simulink model "BC_DC_MotorModel"  (R2022b)
settings: Solver=VariableStepAuto  StartTime=0.0  StopTime=10  RelTol=1e-3
undefined symbols (not defined in the file): b, J, Ke, Kt, L, R
settings Model: Creator=altay  LastModifiedBy=altay

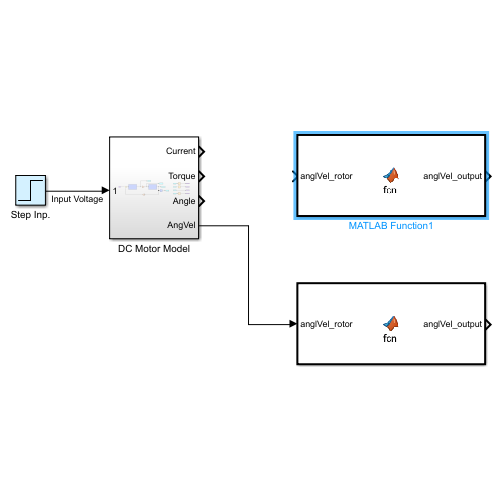
[thumbnail: Simulink's stored preview of the top-level diagram]
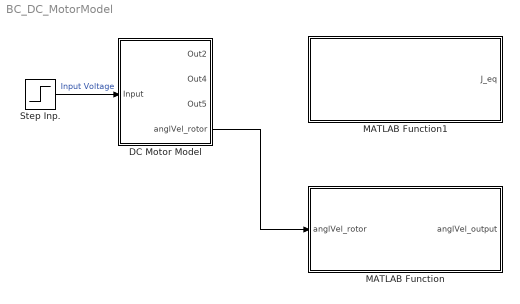
== system BC_DC_MotorModel ==
  DC Motor Model : Subsystem
  MATLAB Function : MATLAB Function  TreatAsAtomicUnit=on
  MATLAB Function1 : MATLAB Function  TreatAsAtomicUnit=on
  Step Inp. : Step  After=250  SampleTime=0
  wires:
  Step Inp./1 -> DC Motor Model/1(Input)  "Input Voltage"
  DC Motor Model/4(anglVel_rotor) -> MATLAB Function/1(anglVel_rotor)

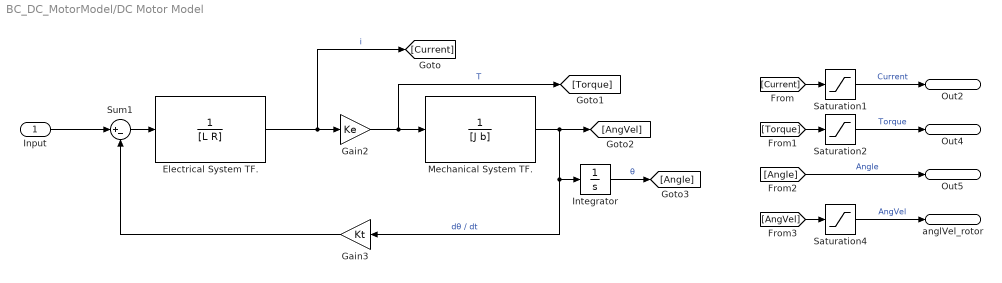
== system BC_DC_MotorModel/DC Motor Model ==
  Input : Inport
  Electrical System TF. : TransferFcn  Denominator=[L R]
  Gain2 : Gain  Gain=Ke
  Gain3 : Gain  Gain=Kt
  Integrator : Integrator
  Mechanical System TF. : TransferFcn  Denominator=[J b]
  Saturation1 : Saturate  UpperLimit=4.87  LowerLimit=-4.87
  Saturation2 : Saturate  UpperLimit=0.105  LowerLimit=-0.105
  Saturation4 : Saturate  UpperLimit=721.519  LowerLimit=-721.519
  Sum1 : Sum  Inputs=|+-
  Out2 : Outport
  Out4 : Outport  Port=2
  Out5 : Outport  Port=3
  anglVel_rotor : Outport  Port=4
  wires:
  Gain2/1 -> [Torque], Mechanical System TF./1  "T"
  Gain3/1 -> Sum1/2
  Electrical System TF./1 -> [Current], Gain2/1  "i"
  Sum1/1 -> Electrical System TF./1
  Input/1 -> Sum1/1
  Mechanical System TF./1 -> [AngVel], Integrator/1, Gain3/1  "dθ / dt"
  Integrator/1 -> [Angle]  "θ"
  Saturation1/1 -> Out2/1  "Current"
  [Current] -> Saturation1/1
  Saturation2/1 -> Out4/1  "Torque"
  [Torque] -> Saturation2/1
  [Angle] -> Out5/1  "Angle"
  Saturation4/1 -> anglVel_rotor/1  "AngVel"
  [AngVel] -> Saturation4/1

== matlab function BC_DC_MotorModel/MATLAB Function ==
  data: anglVel_rotor input; anglVel_output output
function anglVel_output = fcn(anglVel_rotor)
n_values = [21 21 1 70 13 166 12 99];

for x = 1:2:8
    anglVel_output = anglVel_output * n_values(x) / n_values(x + 1);
end

anglVel_output = anglVel_rotor;

== matlab function BC_DC_MotorModel/MATLAB Function1 ==
  data: J_eq output
function J_eq = fcn()
n = [21 21 1 70 13 166 12 99];
J = [1 2 3 4 5 6 7 8];
Jmotor = 10;
Jload = 10;

J_eq = (Jmotor + J(1)) + (J(2)+J(3)) * (n(1)/n(2))^2 + ...
    (J(4) + J(5)) * ((n(1) * n(2)) / n(3) / n(4))^2 + ...
    (J(6) + J(7)) * ((n(1) * n(3) * n(5)) / (n(2) * n(4) * n(6)))^2 + ...
    (J(8) + Jload) * ((n(1) * n(3) * n(5) * n(7)) / (n(2) * n(4) * n(6) * n(8)))^ 2;
